simulink subsystem "MPC16_nlpsol"  (R2022b)
settings: Solver=VariableStepAuto  StartTime=0.0  StopTime=10.0  RelTol=1e-3
undefined symbols (not defined in the file): param_global, param_MPC16, param_robot, param_weight, param_weight_init
settings Model: Creator=emu  LastModifiedBy=emu
settings OptimizationCC: ReuseModelBlockBuffer=on

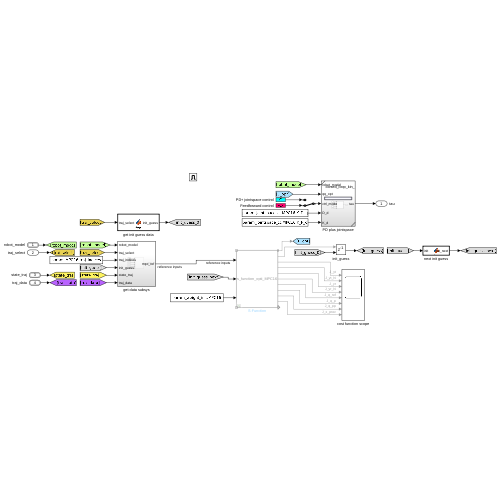
[thumbnail: Simulink's stored preview of the top-level diagram]
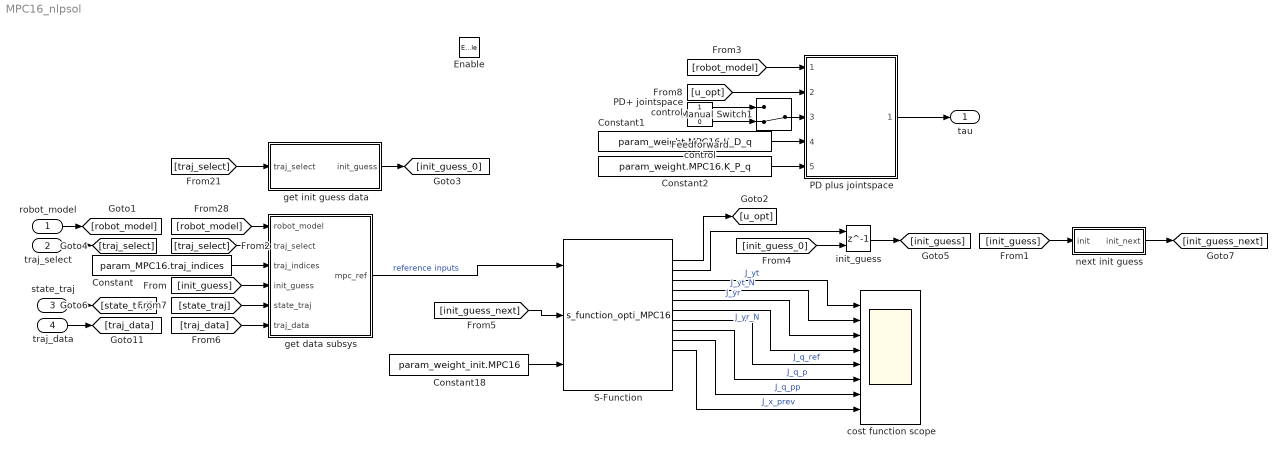
== system MPC16_nlpsol ==
  robot_model : Inport  OutDataTypeStr=Bus: robot_model
  traj_select : Inport  Port=2
  state_traj : Inport  Port=3  OutDataTypeStr=Bus: state_traj_bus
  traj_data : Inport  Port=4  OutDataTypeStr=Bus: traj_data_bus
  Enable : EnablePort
  Constant : Constant  Value=param_MPC16.traj_indices
  Constant1 : Constant  Value=param_weight.MPC16.K_D_q
  Constant18 : Constant  Value=param_weight_init.MPC16  VectorParams1D=off
  Constant2 : Constant  Value=param_weight.MPC16.K_P_q
  Feedforward control : Constant  Value=0
  Manual Switch1 : ManualSwitch  CurrentSetting=0
  PD plus jointspace : Subsystem  ReferencedSubsystem=closed_loop_kin_mpc_pdplus_control_refsys
  PD+ jointspace control : Constant
  S-Function : S-Function  FunctionName=s_function_opti_MPC16  SFunctionModules='MPC16'  SFunctionDeploymentMode=off  EnableBusSupport=off
  cost function scope : Scope  NumInputPorts=8
  get data subsys : Subsystem
  get init guess data : MATLAB Function  TreatAsAtomicUnit=on
  init_guess : Delay  DelayLength=1  InitialConditionSource=Input port  InitialCondition=1  SampleTime=param_global.Ta
      settings: InputPortMap=u0,p4
  next init guess : MATLAB Function  TreatAsAtomicUnit=on
  tau : Outport
  wires:
  Constant/1 -> get data subsys/3(traj_indices)
  [state_traj] -> get data subsys/5(state_traj)
  state_traj/1 -> [state_traj]
  S-Function/2 -> init_guess/1
  [init_guess] -> get data subsys/4(init_guess)
  init_guess/1 -> [init_guess]
  S-Function/1 -> [u_opt]
  S-Function/3 -> cost function scope/1  "J_yt"
  S-Function/5 -> cost function scope/3  "J_yr"
  S-Function/4 -> cost function scope/2  "J_yt_N"
  traj_select/1 -> [traj_select]
  [traj_select] -> get data subsys/2(traj_select)
  [robot_model] -> get data subsys/1(robot_model)
  robot_model/1 -> [robot_model]
  get data subsys/1(mpc_ref) -> S-Function/1  "reference inputs"
  get init guess data/1(init_guess) -> [init_guess_0]
  [traj_select] -> get init guess data/1(traj_select)
  [init_guess_0] -> init_guess/2
  S-Function/6 -> cost function scope/4  "J_yr_N"
  S-Function/7 -> cost function scope/5  "J_q_ref"
  S-Function/8 -> cost function scope/6  "J_q_p"
  next init guess/1(init_next) -> [init_guess_next]
  Constant18/1 -> S-Function/3
  traj_data/1 -> [traj_data]
  [traj_data] -> get data subsys/6(traj_data)
  [init_guess_next] -> S-Function/2
  S-Function/9 -> cost function scope/7  "J_q_pp"
  S-Function/10 -> cost function scope/8  "J_x_prev"
  [init_guess] -> next init guess/1(init)
  PD+ jointspace control/1 -> Manual Switch1/1
  [u_opt] -> PD plus jointspace/2
  Feedforward control/1 -> Manual Switch1/2
  [robot_model] -> PD plus jointspace/1
  Constant2/1 -> PD plus jointspace/5
  Constant1/1 -> PD plus jointspace/4
  Manual Switch1/1 -> PD plus jointspace/3
  PD plus jointspace/1 -> tau/1

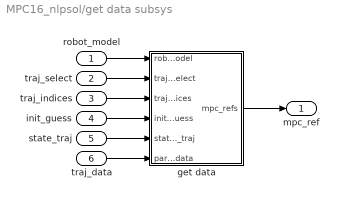
== system MPC16_nlpsol/get data subsys ==
  robot_model : Inport  OutDataTypeStr=Bus: robot_model
  traj_select : Inport  Port=2
  traj_indices : Inport  Port=3
  init_guess : Inport  Port=4
  state_traj : Inport  Port=5  OutDataTypeStr=Bus: state_traj_bus
  traj_data : Inport  Port=6  OutDataTypeStr=Bus: traj_data_bus
  get data : MATLAB Function  TreatAsAtomicUnit=on
  mpc_ref : Outport
  wires:
  traj_data/1 -> get data/6(param_traj_data)
  get data/1(mpc_refs) -> mpc_ref/1
  traj_select/1 -> get data/2(traj_select)
  robot_model/1 -> get data/1(robot_model)
  init_guess/1 -> get data/4(init_guess)
  state_traj/1 -> get data/5(state_traj)
  traj_indices/1 -> get data/3(traj_indices)

== matlab function MPC16_nlpsol/get data subsys/get data ==
  data: robot_model input Bus: robot_model; mpc_refs output; traj_select input; traj_indices input; init_guess input; state_traj input Bus: state_traj_bus; param_robot parameter; param_traj_data input
function mpc_refs   = fcn(robot_model, traj_select, traj_indices, init_guess, state_traj, param_robot, param_traj_data)
persistent cnt;
persistent run_flag;

if(isempty(cnt))
    cnt = 1;
    run_flag = 0;
end

n_red = param_robot.n_red;
n_indices = param_robot.n_indices;

traj_indices = traj_indices + (cnt-1);
N_MPC = length(traj_indices)-1;

% Parameters
q    = robot_model.q;      % generalized coordinates
q_p  = robot_model.q_p;  % time derivative of generalized coordinates

x_k = [q(n_indices);q_p(n_indices)];

% Assemble vector of recieved output measurements
p_d     = param_traj_data.p_d(   1:3, traj_indices, traj_select);
q_d     = param_traj_data.q_d(   1:4, traj_indices, traj_select);

y_d = [p_d; q_d];

%% Reference out
N_u = n_red*N_MPC;
N_x = 2*n_red * (N_MPC+1);

if(cnt == 1)
    u_prev = zeros(N_u,1);
else
    u_prev = init_guess(1:N_u);
end
x_k_prev = init_guess(1+N_u : N_u+N_x);
mpc_refs = [x_k(:); y_d(:); x_k_prev(:); u_prev(:)]';

%% Offline Trajectory out
x_d.p_d            = param_traj_data.p_d(           :,    cnt, traj_select);
x_d.p_d_p          = param_traj_data.p_d_p(         :,    cnt, traj_select);
x_d.p_d_pp         = param_traj_data.p_d_pp(        :,    cnt, traj_select);
x_d.Phi_d          = param_traj_data.Phi_d(         :,    cnt, traj_select);
x_d.Phi_d_p        = param_traj_data.Phi_d_p(       :,    cnt, traj_select);
x_d.Phi_d_pp       = param_traj_data.Phi_d_pp(      :,    cnt, traj_select);
x_d.R_d            = param_traj_data.R_d(           :, :, cnt, traj_select);
x_d.q_d            = param_traj_data.q_d(           :,    cnt, traj_select);
x_d.q_d_p          = param_traj_data.q_d_p(         :,    cnt, traj_select);
x_d.q_d_pp         = param_traj_data.q_d_pp(        :,    cnt, traj_select);
x_d.omega_d        = param_traj_data.omega_d(       :,    cnt, traj_select);
x_d.omega_d_p      = param_traj_data.omega_d_p(     :,    cnt, traj_select);
x_d.alpha_d        = param_traj_data.alpha_d(       :,    cnt, traj_select);
x_d.alpha_d_p      = param_traj_data.alpha_d_p(     :,    cnt, traj_select);
x_d.alpha_d_pp     = param_traj_data.alpha_d_pp(    :,    cnt, traj_select);
x_d.rot_ax_d       = param_traj_data.rot_ax_d(      :,    cnt, traj_select);
x_d.alpha_d_offset = param_traj_data.alpha_d_offset(:,    cnt, traj_select);
x_d.q_d_rel        = param_traj_data.q_d_rel(       :,    cnt, traj_select);

[run_flag, cnt] = update_traj_cnt(state_traj, run_flag, cnt, param_traj_data.N);

== matlab function MPC16_nlpsol/get init guess data ==
  data: traj_select input; param_MPC16_init_guess parameter; init_guess output
function init_guess   = fcn(traj_select, param_MPC16_init_guess)

%init_guess = param_MPC8_init_guess.init_guess(1,:);
init_guess = param_MPC16_init_guess.init_guess(traj_select,:);

== matlab function MPC16_nlpsol/next init guess ==
  data: init input; init_next output; param_MPC16 parameter; param_robot parameter; param_global parameter
function init_next  = fcn(init, param_MPC16, param_robot, param_global)
param_MPC = param_MPC16;

Ta = param_global.Ta;
dt_arr = param_MPC.int_times;
N_MPC = param_MPC.N;
n_red = param_robot.n_red;
N_u = n_red * N_MPC;
N_x = (2*n_red)*(N_MPC+1);

N = 0;

init_next = init';

%% u next
u_idx = N + [1:N_u];       N = N + length(u_idx);
u_idx_2d = reshape(u_idx, n_red, (N_MPC));
u_idx_2d(:, 1:end-1) = u_idx_2d(:, 2:end);
u_init = init(u_idx_2d);

du = (u_init(:, 2:end) - u_init(:, 1:end-1))./dt_arr(1:end-1);
u_next = u_init(:, 1:end-1) + du * Ta;

u_idx_m1 = u_idx_2d(:, 1:end-1);
init_next(u_idx_m1) = u_next;
%% x next
x_idx = N + [1:N_x];       N = N + length(x_idx);
x_idx_2d = reshape(x_idx, 2*n_red, (N_MPC+1));
x_idx_2d(:, 1:end-1) = x_idx_2d(:, 2:end);
x_init = init(x_idx_2d);

dx = (x_init(:, 2:end) - x_init(:, 1:end-1))./dt_arr;
x_next = x_init(:, 1:end-1) + dx * Ta;

x_idx_m1 = x_idx_2d(:, 1:end-1);
init_next(x_idx_m1) = x_next;
